simulink model "Simimplement"  (R2021b)
settings: Solver=VariableStepAuto  StartTime=0.0  StopTime=10.0  RelTol=1e-3
model workspace (MAT data in the model file):
  K_c = 15
values from neighbouring files (symbols this model uses):
  A = [-(L_Alpha/(U_0*m)) U_0 0; (L_Alpha*l_Alpha)/(U_0*I_y) 0  0;  0 1 0]    [Simulinkimplement.m]
  B = [(T_c/m); ((l_c*T_c)/I_y); 0]    [Simulinkimplement.m]
  C = eye(3,3)    [Simulinkimplement.m]
  D = zeros(3,1)    [Simulinkimplement.m]
  delta_max = delta_max_deg*pi/180    (= 0.174532925199)    [Simulinkimplement.m]    (also in Simulinkimplement152.m; Simulinkimplement72.m)
  K_A = 6    [Simulinkimplement.m]    (also in Simulinkimplement152.m = 6.8; Simulinkimplement72.m = 52)
  K_R = 0.5    [Simulinkimplement.m]    (also in Simulinkimplement152.m; Simulinkimplement72.m; Task1.m = 0.3; Task1time152sec.m = 0.3)
  theta_c = theta_c_deg*pi/180    (= 0.0872664625997)    [Simulinkimplement.m]    (also in Simulinkimplement152.m; Simulinkimplement72.m)
settings Model: Creator=raghu  LastModifiedBy=raghu
settings SolverCC: AlgebraicLoopSolver=TrustRegion
settings DebuggingCC: SFMachineParentedDataDiag=warning

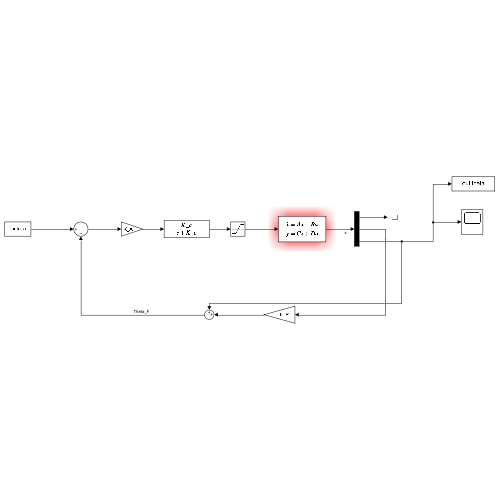
[thumbnail: Simulink's stored preview of the top-level diagram]
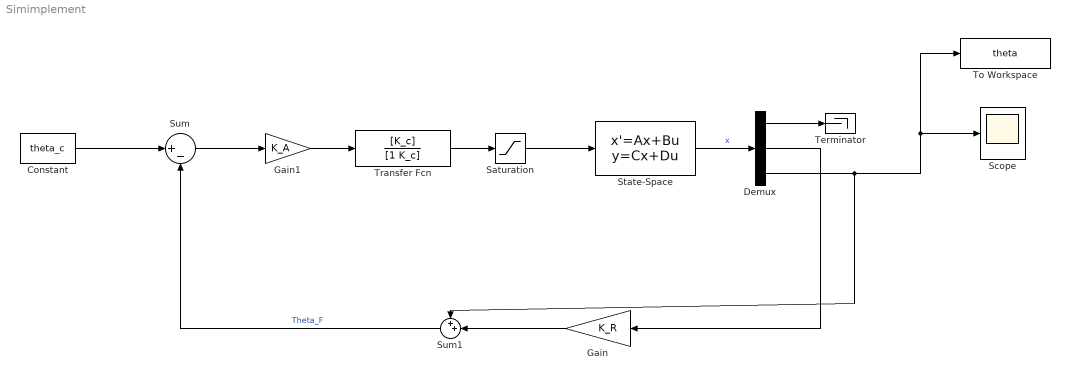
== system Simimplement ==
  Constant : Constant  Value=theta_c
  Demux : Demux  Outputs=3
  Gain : Gain  Gain=K_R
  Gain1 : Gain  Gain=K_A
  Saturation : Saturate  UpperLimit=delta_max  LowerLimit=-delta_max
  Scope : Scope
  State-Space : StateSpace  A=A  B=B  C=C  D=D  InitialCondition=0
  Sum : Sum  Inputs=|+-
  Sum1 : Sum  Inputs=++|
  Terminator : Terminator
  To Workspace : ToWorkspace  VariableName=theta  SaveFormat=Timeseries  SampleTime=-1
  Transfer Fcn : TransferFcn  Numerator=[K_c]  Denominator=[1 K_c]
  wires:
  Constant/1 -> Sum/1
  State-Space/1 -> Demux/1  "x"
  Demux/2 -> Gain/1
  Demux/3 -> To Workspace/1, Scope/1, Sum1/1
  Gain/1 -> Sum1/2
  Sum1/1 -> Sum/2  "Theta_F"
  Demux/1 -> Terminator/1
  Sum/1 -> Gain1/1
  Gain1/1 -> Transfer Fcn/1
  Transfer Fcn/1 -> Saturation/1
  Saturation/1 -> State-Space/1
